simulink model "Torque_Vectoring_Schanzer20"  (R2018a)
settings: Solver=ode15s  StartTime=0.01  StopTime=inf  RelTol=1e-3  EnableMultiTasking=on
libraries: CarMaker4SL x8, dspstat3 x5, simulink x2
(part 3 of 3)

== system Torque_Vectoring_Schanzer20/CarMaker/IPG Vehicle/PowerTrain/Torque Vectoring System/Controller Logic1/Torque Vectoring/torque distribution/feedback control ==
  desired Yaw rate rad/s : Inport
  yaw rate sensor : Inport  Port=2
  ratioF : Inport  Port=3
  ratioR : Inport  Port=4
  twidth F : Inport  Port=5
  twidth R : Inport  Port=6
  Abs : Abs
  Divide1 : Product  Inputs=*/
  Divide2 : Product  Inputs=*/
  Gain : Gain  Gain=5.6
  Gain1 : Gain  Gain=12.8
  Gain2 : Gain  Gain=12.8
  Median Filter : dspstat3/Median Filter  WindowLength=100  SimulateUsing=Interpreted execution
      settings: SourceProductName=DSP System Toolbox  SourceProductBaseCode=DS
  Multiply : Product
  Multiply1 : Product
  PID Controller : simulink/Continuous/PID Controller  Controller=PID  TimeDomain=Continuous-time  SampleTime=-1  IntegratorMethod=Forward Euler  FilterMethod=Forward Euler  Form=Parallel  UseFilter=on  ControllerParametersSource=internal  P=53.9348  I=3.159  D=0  N=0  InitialConditionSource=internal  InitialConditionForIntegrator=0  InitialConditionForFilter=0  ExternalReset=none  LimitOutput=on  UpperSaturationLimit=550  LowerSaturationLimit=-550  LinearizeAsGain=off  AntiWindupMode=none  Kb=1  TrackingMode=off  Kt=1  PParamMin=[]  PParamMax=[]  IParamMin=[]  IParamMax=[]  DParamMin=[]  DParamMax=[]  NParamMin=[]  NParamMax=[]  KbParamMin=[]  KbParamMax=[]  KtParamMin=[]  KtParamMax=[]  POutMin=[]  POutMax=[]  IOutMin=[]  IOutMax=[]  DOutMin=[]  DOutMax=[]  NOutMin=[]  NOutMax=[]  KbOutMin=[]  KbOutMax=[]  KtOutMin=[]  KtOutMax=[]  IntegratorOutMin=[]  IntegratorOutMax=[]  FilterOutMin=[]  FilterOutMax=[]  SumOutMin=[]  SumOutMax=[]  SumI1OutMin=[]  SumI1OutMax=[]  SumI2OutMin=[]  SumI2OutMax=[]  SumI3OutMin=[]  SumI3OutMax=[]  SumDOutMin=[]  SumDOutMax=[]  SaturationOutMin=[]  SaturationOutMax=[]  IntegratorContinuousStateAttributes=''  IntegratorStateMustResolveToSignalObject=off  IntegratorRTWStateStorageClass=Auto  FilterContinuousStateAttributes=''  FilterStateMustResolveToSignalObject=off  FilterRTWStateStorageClass=Auto  DifferentiatorICPrevScaledInput=0  DifferentiatorOutMin=[]  DifferentiatorOutMax=[]  FilterDiffOutCoefMin=[]  FilterDiffOutCoefMax=[]  SumDenOutMin=[]  SumDenOutMax=[]  SumNumOutMin=[]  SumNumOutMax=[]  ReciprocalOutMin=[]  ReciprocalOutMax=[]  DivideOutMin=[]  DivideOutMax=[]  TunerSelectOption=Transfer Function Based (PID Tuner App)
  Scope : Scope  NumInputPorts=2
  Sum : Sum  Inputs=-+
  Switch : Switch  Criteria=u2 > Threshold  Threshold=0.02
  Tfront : Outport
  Trear : Outport  Port=2
  yaw sensor : Outport  Port=3
  wires:
  PID Controller/1 -> Multiply1/1, Multiply/1  "saturation output"
  desired Yaw rate rad/s/1 -> Gain/1  "reference yaw rate"
  Abs/1 -> Switch/2
  Median Filter/1 -> Switch/1, Abs/1
  Switch/1 -> Scope/1, yaw sensor/1  "Sensor Yaw Rate"
  Gain/1 -> Scope/2, Sum/2  "Target Yaw Rate"
  Sum/1 -> PID Controller/1
  Gain2/1 -> Trear/1
  twidth F/1 -> Divide1/2
  Gain1/1 -> Tfront/1
  Divide1/1 -> Gain1/1
  twidth R/1 -> Divide2/2
  Divide2/1 -> Gain2/1
  ratioF/1 -> Multiply/2
  ratioR/1 -> Multiply1/2
  Multiply/1 -> Divide1/1
  Multiply1/1 -> Divide2/1
  yaw rate sensor/1 -> Sum/1, Median Filter/1
